simulink model "chap3_4sim"  (Simulink 6.3)
settings: Solver=ode45  StartTime=0.0  StopTime=2000  RelTol=1e-3
libraries: simulink x1, simulink_extras x1
settings Model: Creator=hp  LastModifiedBy=Administrator  ExtModeTrigMode=oneshot  ExtModeArmWhenConnect=off
settings DataIOCC: LimitDataPoints=off  SignalLoggingName=sigsOut
settings OptimizationCC: BooleanDataType=off
settings DebuggingCC: SolverPrmCheckMsg=none
settings HardwareCC: TargetUnknown=on

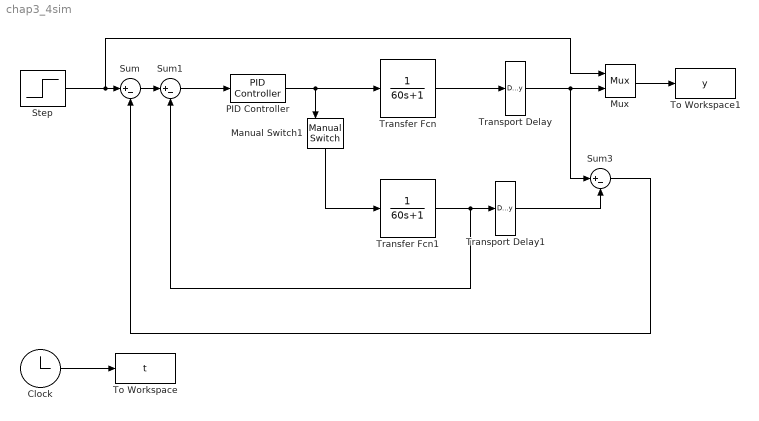
== system chap3_4sim ==
  Clock : Clock
      settings: Decimation=10
  Manual Switch1 : simulink/Signal Routing/Manual Switch  Orientation=down  sw=1  action=0
  Mux : Mux  Inputs=2
  PID Controller : simulink_extras/Additional Linear/PID Controller  P=4  I=0.022  D=0.0
  Step : Step  Time=0  After=100  SampleTime=0
  Sum : Sum  Inputs=|+-  SaturateOnIntegerOverflow=on  InputSameDT=on
  Sum1 : Sum  Inputs=|+-  SaturateOnIntegerOverflow=on  InputSameDT=on
  Sum3 : Sum  Inputs=|+-  SaturateOnIntegerOverflow=on  InputSameDT=on
  To Workspace : ToWorkspace  VariableName=t  SampleTime=-1  SaveFormat=Array
  To Workspace1 : ToWorkspace  VariableName=y  SampleTime=-1  SaveFormat=Array
  Transfer Fcn : TransferFcn  Denominator=[60 1]
  Transfer Fcn1 : TransferFcn  Denominator=[60 1]
  Transport Delay : TransportDelay  DelayTime=80
  Transport Delay1 : TransportDelay  DelayTime=80
  wires:
  PID Controller/1 -> Transfer Fcn/1, Manual Switch1/1
  Sum/1 -> Sum1/1
  Step/1 -> Mux/1, Sum/1
  Sum1/1 -> PID Controller/1
  Transfer Fcn/1 -> Transport Delay/1
  Transport Delay/1 -> Mux/2, Sum3/1
  Mux/1 -> To Workspace1/1
  Transfer Fcn1/1 -> Transport Delay1/1, Sum1/2
  Transport Delay1/1 -> Sum3/2
  Clock/1 -> To Workspace/1
  Sum3/1 -> Sum/2
  Manual Switch1/1 -> Transfer Fcn1/1
